simulink model "pr4"  (R2020a)
settings: Solver=FixedStepDiscrete  StartTime=0.0  StopTime=20.0  FixedStep=1  RelTol=1e-3
settings Model: Creator=Admin  LastModifiedBy=Admin

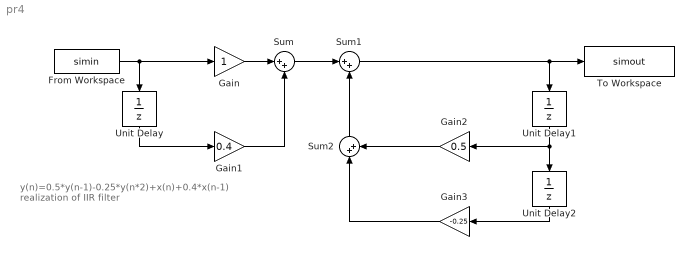
== system pr4 ==
  note: y(n)=0.5*y(n-1)-0.25*y(n*2)+x(n)+0.4*x(n-1)
      | realization of IIR filter
  From Workspace : FromWorkspace  VariableName=simin
  Gain : Gain
  Gain1 : Gain  Gain=0.4
  Gain2 : Gain  Gain=0.5
  Gain3 : Gain  Gain=-0.25
  Sum : Sum  Inputs=|++
  Sum1 : Sum  Inputs=|++
  Sum2 : Sum  Inputs=|++
  To Workspace : ToWorkspace  VariableName=simout  SaveFormat=Timeseries  SampleTime=-1
  Unit Delay : UnitDelay  SampleTime=-1  HasFrameUpgradeWarning=on
  Unit Delay1 : UnitDelay  SampleTime=-1  HasFrameUpgradeWarning=on
  Unit Delay2 : UnitDelay  SampleTime=-1  HasFrameUpgradeWarning=on
  wires:
  From Workspace/1 -> Gain/1, Unit Delay/1
  Unit Delay/1 -> Gain1/1
  Gain/1 -> Sum/1
  Gain1/1 -> Sum/2
  Sum/1 -> Sum1/1
  Sum1/1 -> Unit Delay1/1, To Workspace/1
  Unit Delay1/1 -> Gain2/1, Unit Delay2/1
  Unit Delay2/1 -> Gain3/1
  Sum2/1 -> Sum1/2
  Gain2/1 -> Sum2/2
  Gain3/1 -> Sum2/1
